simulink model "trialnew"  (R2019a)
settings: Solver=VariableStepAuto  StartTime=0.0  StopTime=10.0  RelTol=1e-3
libraries: truetime x5
settings Model: Creator=Dell  LastModifiedBy=Dell

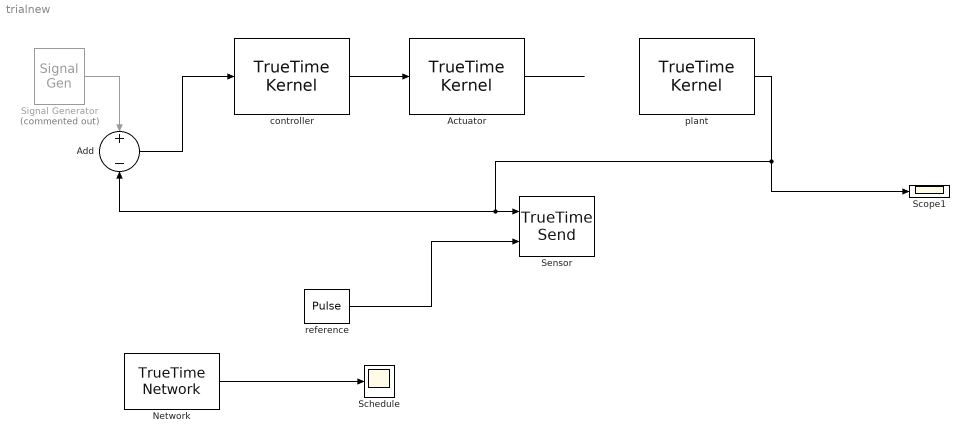
== system trialnew ==
  "Actuator " : truetime/TrueTime Kernel  sfun=actuator_init  args=[]  ninputsoutputs=[1 0]  ntriggers=0  trigtype=falling  nwnodenbr=[]  clockoffsetdrift=[0 0]  schedoutput=on  battery=off  poweroutput=off
  Add : Sum  Inputs=+-
  Network : truetime/TrueTime Network  nwtype=CSMA/CD (Ethernet)  nwnbr=1  nnodes=1  rate=10000000  minsize=512  lossprob=0  seed=0  bandwidths=[0.5 0.5]  slotsize=512  schedule=[1 1 2]  memsize=80000  buftype=Common buffer  overflow=Retransmit  dynSchedule=0  miniSlotSize=0  NIT=0  QSortMode=FIFO  sync=0  irtSchedule=0  nrtLength=0  nodeGraph=0  scheduleoutput=on
  "Schedule " : Scope
  Scope1 : Scope
  Sensor : truetime/TrueTime Send  trigger=falling  nwnbr=1  sender=1  indim=1  recsource=internal  receiver=1  lengthsource=internal  length=1000  priosource=internal  prio=1  msgIDsource=internal  msgID=0  dynamicSegment=dynamic
  Signal Generator : SignalGenerator  Commented=on  Units=rad/sec
  controller : truetime/TrueTime Kernel  sfun=node_init  args=[]  ninputsoutputs=[1 0]  ntriggers=0  trigtype=falling  nwnodenbr=[]  clockoffsetdrift=[0 0]  schedoutput=on  battery=off  poweroutput=off
  plant : truetime/TrueTime Kernel  sfun=node_init  args=[]  ninputsoutputs=[1 0]  ntriggers=0  trigtype=falling  nwnodenbr=[]  clockoffsetdrift=[0 0]  schedoutput=on  battery=off  poweroutput=off
  reference : DiscretePulseGenerator  PulseType=Time based  Period=1.2  PulseWidth=50
  wires:
  reference/1 -> Sensor/2
  Network/1 -> "Schedule "/1
  plant/1 -> Scope1/1, Add/2, Sensor/1
  Signal Generator/1 -> Add/1
  controller/1 -> "Actuator "/1
  Add/1 -> controller/1
  "Actuator "/1 -> ?
  ? -> plant/1
